simulink model "CRA_Assignment4"  (R2022b)
settings: Solver=ode23  StartTime=0.0  StopTime=200  RelTol=1e-7  AbsTol=1e-7
settings Model: Creator=lerio  LastModifiedBy=lerio

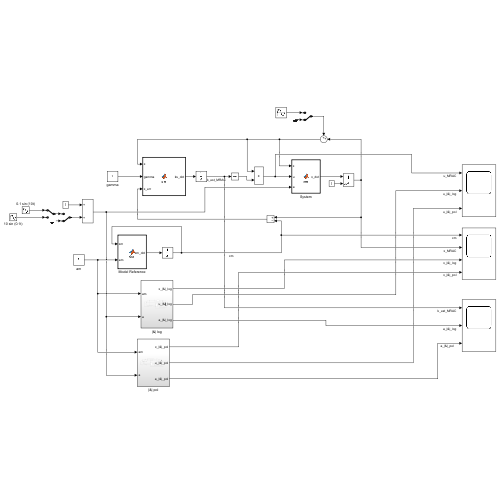
[thumbnail: Simulink's stored preview of the top-level diagram]
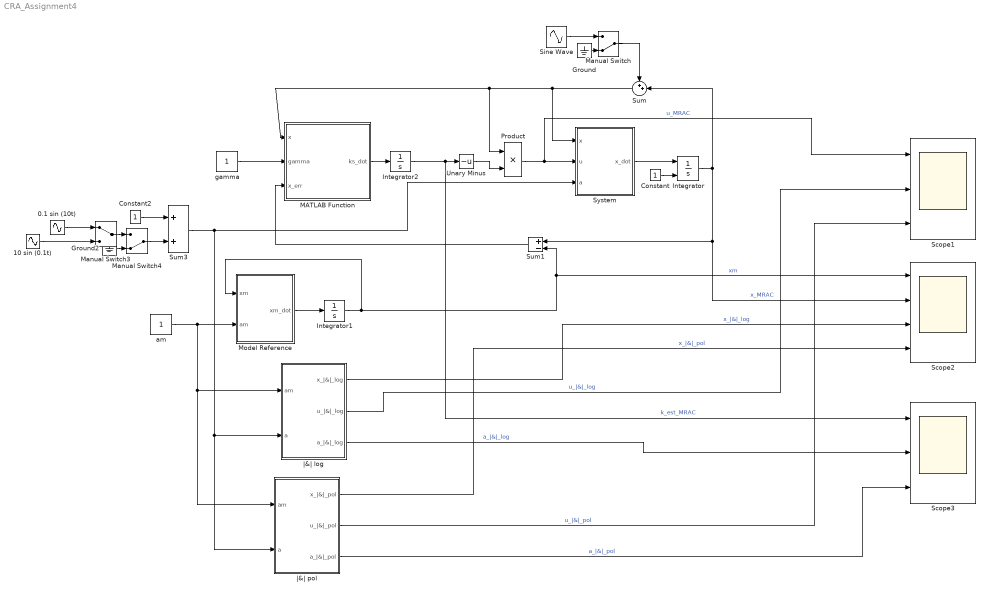
== system CRA_Assignment4 ==
  0.1 sin (10t) : Sin  Amplitude=0.1  Frequency=10  SampleTime=0
  10 sin (0.1t) : Sin  Amplitude=10  Frequency=0.1  SampleTime=0
  Constant : Constant
  Constant2 : Constant
  Ground : Ground
  Ground2 : Ground
  Integrator : Integrator  InitialConditionSource=external
  Integrator1 : Integrator
  Integrator2 : Integrator
  MATLAB Function : MATLAB Function  TreatAsAtomicUnit=on
  Manual Switch : ManualSwitch  CurrentSetting=0
  Manual Switch3 : ManualSwitch
  Manual Switch4 : ManualSwitch  CurrentSetting=0
  Model Reference : MATLAB Function  TreatAsAtomicUnit=on
  Product : Product
  Scope1 : Scope  NumInputPorts=3
  Scope2 : Scope  NumInputPorts=4
  Scope3 : Scope  NumInputPorts=3
  Sine Wave : Sin  Amplitude=0.5  Frequency=0.20  SampleTime=0
  Sum : Sum  Inputs=++|
  Sum1 : Sum  Inputs=+-
  Sum3 : Sum
  System : MATLAB Function  TreatAsAtomicUnit=on
  Unary Minus : UnaryMinus
  am : Constant
  gamma : Constant
  |&| log : Subsystem
  |&| pol : Subsystem
  wires:
  System/1(x_dot) -> Integrator/1
  Integrator/1 -> Scope2/2, Sum1/1, Sum/2  "x_MRAC"
  Integrator1/1 -> Sum1/2, Scope2/1, Model Reference/1(xm)  "xm"
  Model Reference/1(xm_dot) -> Integrator1/1
  Sum1/1 -> MATLAB Function/3(x_err)
  gamma/1 -> MATLAB Function/2(gamma)
  MATLAB Function/1(ks_dot) -> Integrator2/1
  Integrator2/1 -> Scope3/1, Unary Minus/1  "k_est_MRAC"
  Unary Minus/1 -> Product/2
  Product/1 -> System/2(u), Scope1/1  "u_MRAC"
  am/1 -> |&| pol/1(am), |&| log/1(am), Model Reference/2(am)
  Constant/1 -> Integrator/2
  |&| log/1(x_|&|_log) -> Scope2/3  "x_|&|_log"
  |&| pol/1(x_|&|_pol) -> Scope2/4  "x_|&|_pol"
  |&| log/2(u_|&|_log) -> Scope1/2  "u_|&|_log"
  |&| pol/2(u_|&|_pol) -> Scope1/3  "u_|&|_pol"
  |&| pol/3(a_|&|_pol) -> Scope3/3  "a_|&|_pol"
  |&| log/3(a_|&|_log) -> Scope3/2  "a_|&|_log"
  Sum/1 -> System/1(x), Product/1, MATLAB Function/1(x)
  Sine Wave/1 -> Manual Switch/1
  Ground/1 -> Manual Switch/2
  Manual Switch/1 -> Sum/1
  0.1 sin (10t)/1 -> Manual Switch3/1
  10 sin (0.1t)/1 -> Manual Switch3/2
  Manual Switch3/1 -> Manual Switch4/1
  Manual Switch4/1 -> Sum3/2
  Constant2/1 -> Sum3/1
  Ground2/1 -> Manual Switch4/2
  Sum3/1 -> |&| log/2(a), |&| pol/2(a), System/3(a)

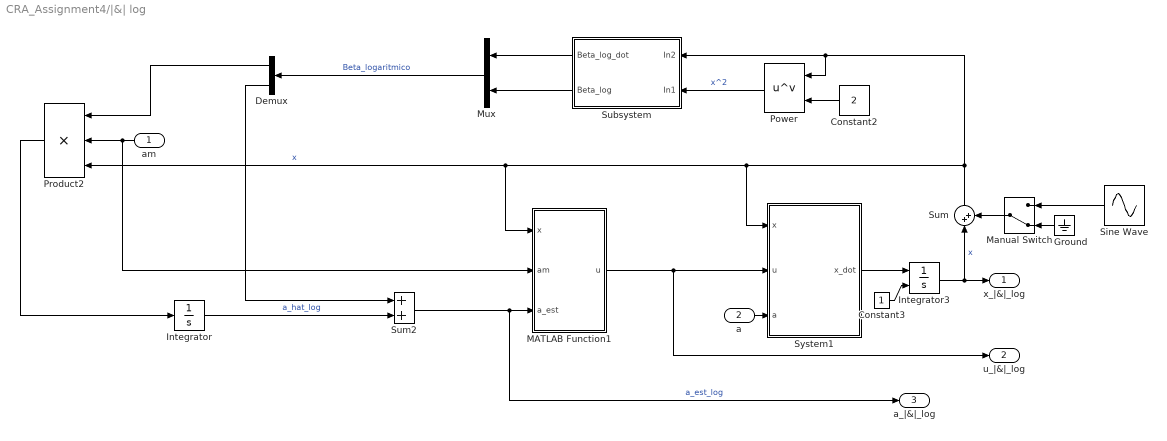
== system CRA_Assignment4/|&| log ==
  am : Inport
  a : Inport  Port=2
  Constant2 : Constant  Value=2
  Constant3 : Constant
  Demux : Demux  Outputs=2
  Ground : Ground
  Integrator : Integrator
  Integrator3 : Integrator  InitialConditionSource=external
  MATLAB Function1 : MATLAB Function  TreatAsAtomicUnit=on
  Manual Switch : ManualSwitch  CurrentSetting=0
  Mux : Mux  Inputs=2
  Power : Math  Operator=pow
  Product2 : Product  Inputs=3
  Sine Wave : Sin  Amplitude=0.5  Frequency=0.20  SampleTime=0
  Subsystem : Subsystem
  Sum : Sum  Inputs=|++
  Sum2 : Sum
  System1 : MATLAB Function  TreatAsAtomicUnit=on
  x_|&|_log : Outport
  u_|&|_log : Outport  Port=2
  a_|&|_log : Outport  Port=3
  wires:
  Constant3/1 -> Integrator3/2
  System1/1(x_dot) -> Integrator3/1
  Mux/1 -> Demux/1  "Beta_logaritmico"
  Integrator3/1 -> Sum/1, x_|&|_log/1  "x"
  Demux/2 -> Sum2/1
  Subsystem/2(Beta_log) -> Mux/2
  Demux/1 -> Product2/1
  Constant2/1 -> Power/2
  Subsystem/1(Beta_log_dot) -> Mux/1
  Power/1 -> Subsystem/2(In1)  "x^2"
  am/1 -> MATLAB Function1/2(am), Product2/2
  Product2/1 -> Integrator/1
  Integrator/1 -> Sum2/2  "a_hat_log"
  Sum2/1 -> a_|&|_log/1, MATLAB Function1/3(a_est)  "a_est_log"
  MATLAB Function1/1(u) -> u_|&|_log/1, System1/2(u)
  Sum/1 -> System1/1(x), MATLAB Function1/1(x), Product2/3, Power/1, Subsystem/1(In2)  "x"
  Manual Switch/1 -> Sum/2
  Ground/1 -> Manual Switch/2
  Sine Wave/1 -> Manual Switch/1
  a/1 -> System1/3(a)

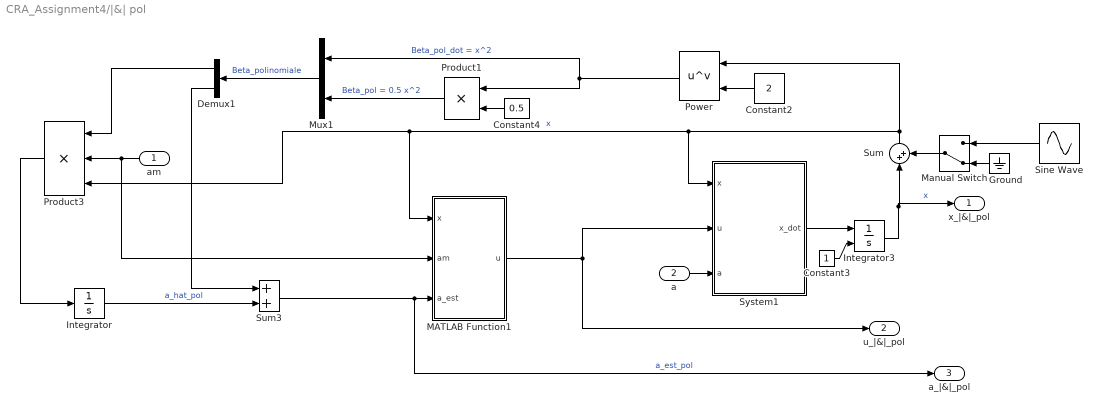
== system CRA_Assignment4/|&| pol ==
  am : Inport
  a : Inport  Port=2
  Constant2 : Constant  Value=2
  Constant3 : Constant
  Constant4 : Constant  Value=0.5
  Demux1 : Demux  Outputs=2
  Ground : Ground
  Integrator : Integrator
  Integrator3 : Integrator  InitialConditionSource=external
  MATLAB Function1 : MATLAB Function  TreatAsAtomicUnit=on
  Manual Switch : ManualSwitch  CurrentSetting=0
  Mux1 : Mux  Inputs=2
  Power : Math  Operator=pow
  Product1 : Product
  Product3 : Product  Inputs=3
  Sine Wave : Sin  Amplitude=0.5  Frequency=0.20  SampleTime=0
  Sum : Sum  Inputs=|++
  Sum3 : Sum
  System1 : MATLAB Function  TreatAsAtomicUnit=on
  x_|&|_pol : Outport
  u_|&|_pol : Outport  Port=2
  a_|&|_pol : Outport  Port=3
  wires:
  Constant3/1 -> Integrator3/2
  Integrator3/1 -> Sum/1, x_|&|_pol/1  "x"
  Constant2/1 -> Power/2
  System1/1(x_dot) -> Integrator3/1
  Demux1/2 -> Sum3/1
  Demux1/1 -> Product3/1
  Product1/1 -> Mux1/2  "Beta_pol = 0.5 x^2"
  Mux1/1 -> Demux1/1  "Beta_polinomiale"
  Power/1 -> Product1/1, Mux1/1  "Beta_pol_dot = x^2"
  Constant4/1 -> Product1/2
  am/1 -> MATLAB Function1/2(am), Product3/2
  Product3/1 -> Integrator/1
  Integrator/1 -> Sum3/2  "a_hat_pol"
  Sum3/1 -> a_|&|_pol/1, MATLAB Function1/3(a_est)  "a_est_pol"
  MATLAB Function1/1(u) -> u_|&|_pol/1, System1/2(u)
  Ground/1 -> Manual Switch/2
  Manual Switch/1 -> Sum/2
  Sine Wave/1 -> Manual Switch/1
  Sum/1 -> Power/1, System1/1(x), MATLAB Function1/1(x), Product3/3  "x"
  a/1 -> System1/3(a)

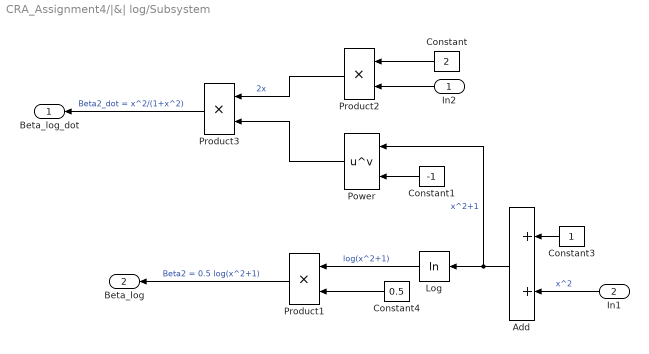
== system CRA_Assignment4/|&| log/Subsystem ==
  In2 : Inport
  In1 : Inport  Port=2
  Add : Sum
  Constant : Constant  Value=2
  Constant1 : Constant  Value=-1
  Constant3 : Constant
  Constant4 : Constant  Value=0.5
  Log : Math  Operator=log
  Power : Math  Operator=pow
  Product1 : Product
  Product2 : Product
  Product3 : Product
  Beta_log_dot : Outport
  Beta_log : Outport  Port=2
  wires:
  Product1/1 -> Beta_log/1  "Beta2 = 0.5 log(x^2+1)"
  Log/1 -> Product1/1  "log(x^2+1)"
  Constant3/1 -> Add/1
  In1/1 -> Add/2  "x^2"
  Add/1 -> Power/1, Log/1  "x^2+1"
  Constant4/1 -> Product1/2
  Constant/1 -> Product2/1
  In2/1 -> Product2/2
  Constant1/1 -> Power/2
  Power/1 -> Product3/2
  Product2/1 -> Product3/1  "2x"
  Product3/1 -> Beta_log_dot/1  "Beta2_dot = x^2/(1+x^2)"

== matlab function CRA_Assignment4/System ==
  data: x input; u input; x_dot output; a input
function x_dot = fcn(x,u,a)

x_dot = a*x+u;

== matlab function CRA_Assignment4/MATLAB Function ==
  data: x input; gamma input; x_err input; ks_dot output
function ks_dot = fcn(x, gamma, x_err)

ks_dot = gamma*x_err*x;

== matlab function CRA_Assignment4/|&| log/MATLAB Function1 ==
  data: x input; am input; a_est input; u output
function u = fcn(x,am,a_est)

u = -am*x - a_est*x;

== matlab function CRA_Assignment4/|&| log/System1 ==
  data: x input; u input; x_dot output; a input
function x_dot = fcn(x,u,a)

x_dot = a*x+u;

== matlab function CRA_Assignment4/|&| pol/System1 ==
  data: x input; u input; x_dot output; a input
function x_dot = fcn(x,u,a)

x_dot = a*x+u;

== matlab function CRA_Assignment4/|&| pol/MATLAB Function1 ==
  data: x input; am input; a_est input; u output
function u = fcn(x,am,a_est)

u = -am*x - a_est*x;

== matlab function CRA_Assignment4/Model Reference ==
  data: xm input; xm_dot output; am input
function xm_dot = fcn(xm,am)

xm_dot = -am*xm;
